simulink model "AIM_OneAgent"  (R2022b)
settings: Solver=ode4  StartTime=0.0  StopTime=inf  FixedStep=0.01  RelTol=1e-3
libraries: simulink x6, slpidlib x4, sim3dautolib x4, rllib x2, sim3dlib x1
(part 1 of 2)
settings Model: Creator=DELL G3  LastModifiedBy=DELL G3
settings DebuggingCC: IgnoredZcDiagnostic=none

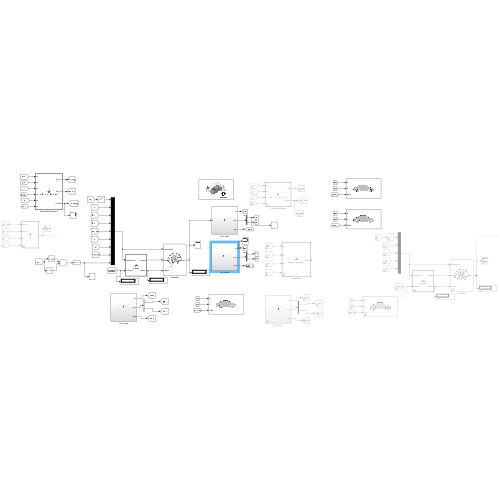
[thumbnail: Simulink's stored preview of the top-level diagram]
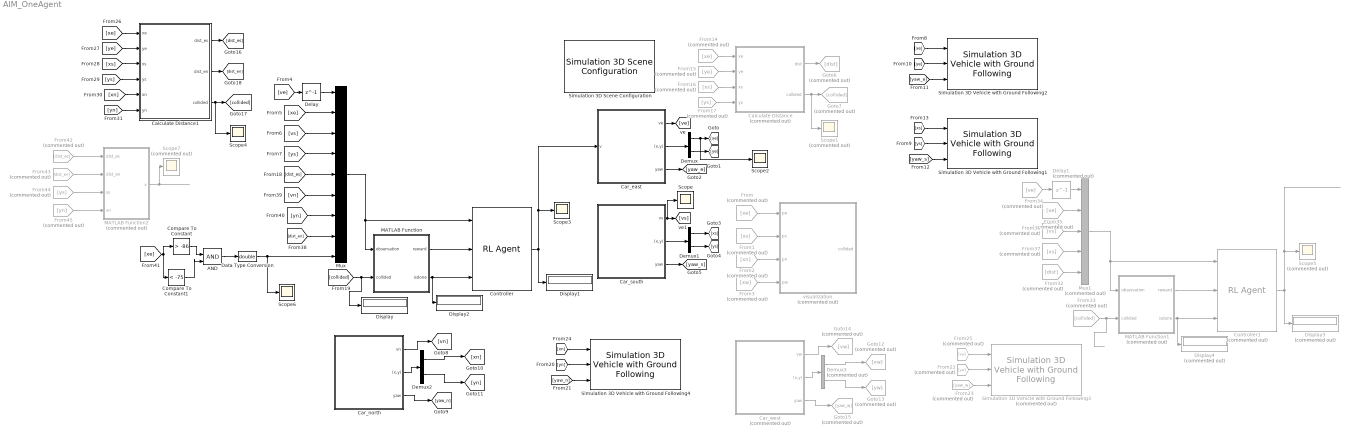
== system AIM_OneAgent ==
  AND : Logic  IconShape=distinctive  AllPortsSameDT=off  OutDataTypeStr=boolean
  Calculate Distance : MATLAB Function  Commented=on  TreatAsAtomicUnit=on
  Calculate Distance1 : MATLAB Function  TreatAsAtomicUnit=on
  Car_east : Subsystem
  Car_north : Subsystem
  Car_south : Subsystem
  Car_west : Subsystem  Commented=on
  Compare To Constant : simulink/Logic and Bit Operations/Compare To Constant  relop=>  const=-86  OutDataTypeStr=boolean
  Compare To Constant1 : simulink/Logic and Bit Operations/Compare To Constant  relop=<  const=-75  OutDataTypeStr=boolean
  Controller : rllib/RL Agent  Agent=car_agent_Trained  ExternalActionAsInput=off  ProvideLastAction=off  ProvideCumRwd=off  TreatAsDirectFeedthrough=on  UseStrictObservationDataTypes=off
  Controller1 : rllib/RL Agent  Commented=on  Agent=agent1_Trained_Trained  ExternalActionAsInput=off  ProvideLastAction=off  ProvideCumRwd=off  TreatAsDirectFeedthrough=on  UseStrictObservationDataTypes=off
  Data Type Conversion : DataTypeConversion  OutDataTypeStr=double  SaturateOnIntegerOverflow=off  RndMeth=Floor
  Delay : Delay  DelayLength=1
  Delay1 : Delay  Commented=on  DelayLength=1
  Demux : Demux  Outputs=2
  Demux1 : Demux  Outputs=2
  Demux2 : Demux  Outputs=2
  Demux3 : Demux  Commented=on  Outputs=2
  Display : Display
  Display1 : Display
  Display2 : Display
  Display3 : Display  Commented=on
  Display4 : Display  Commented=on
  From : From  Commented=on  GotoTag=xe
  From1 : From  Commented=on  GotoTag=xs
  From14 : From  Commented=on  GotoTag=xe
  From15 : From  Commented=on  GotoTag=ye
  From16 : From  Commented=on  GotoTag=xs
  From17 : From  Commented=on  GotoTag=ys
  From2 : From  Commented=on  GotoTag=xn
  From22 : From  Commented=on  GotoTag=yw
  From23 : From  Commented=on  GotoTag=yaw_w
  From25 : From  Commented=on  GotoTag=xw
  From3 : From  Commented=on  GotoTag=xw
  From32 : From  Commented=on  GotoTag=dist
  From33 : From  Commented=on  GotoTag=collided
  From34 : From  Commented=on  GotoTag=ve
  From35 : From  Commented=on  GotoTag=xe
  From36 : From  Commented=on  GotoTag=vs
  From37 : From  Commented=on  GotoTag=xs
  From42 : From  Commented=on  GotoTag=dist_es
  From43 : From  Commented=on  GotoTag=dist_en
  From44 : From  Commented=on  GotoTag=ys
  From45 : From  Commented=on  GotoTag=yn
  Goto12 : Goto  Commented=on  GotoTag=xw
  Goto13 : Goto  Commented=on  GotoTag=yw
  Goto14 : Goto  Commented=on  GotoTag=vw
  Goto15 : Goto  Commented=on  GotoTag=yaw_w
  Goto6 : Goto  Commented=on  GotoTag=dist
  Goto7 : Goto  Commented=on  GotoTag=collided
  MATLAB Function : MATLAB Function  TreatAsAtomicUnit=on
  MATLAB Function1 : MATLAB Function  Commented=on  TreatAsAtomicUnit=on
  MATLAB Function2 : MATLAB Function  Commented=on  TreatAsAtomicUnit=on
  Mux : Mux  Inputs=9
  Mux1 : Mux  Commented=on  Inputs=5
  Scope{,2..4,6} (5 alike) : Scope
  Scope1 : Scope  Commented=on
  Scope5 : Scope  Commented=on
  Scope7 : Scope  Commented=on
  Simulation 3D Scene Configuration : sim3dlib/Simulation 3D Scene Configuration  Priority=0  ProjectFormat=Default Scenes  SceneDesc=US city block  ProjectName=C:\Program Files\MATLAB\R2022b\toolbox\shared\sim3d_projects\automotive_project\UE4\WindowsNoEditor\VehicleSimulation.exe  ScenePath=/Game/Maps/HwStrght  EnableOpenDRIVE=off  vehTagList={'Scene Origin';'car_east';'car_north';'car_south';'car_west'}  vehTag=car_east  OpVisEn=off  Ts=0.01  EnableWindow=on  EnableRemoteAccess=off  EnableWeather=off  SunAltitude=40.0  SunAzimuth=90  clouds=10  wind=1  fog=0  rain=0  EnableGeospatial=off  OriginHeight=200  OriginLatitude=40.744652  OriginLongitude=-73.988864  MapStyle=Aerial  AdditionalAssetIDs=[]  UseAdvancedSunSky=off  SolarTime=11  TimeZone=-5  Day=21  Month=9  Year=2022  UseDaylightSavingTime=on  DSTStartDay=10  DSTStartMonth=3  DSTEndDay=3  DSTEndMonth=11  DSTSwitchHour=2  sensorTag=MainCamera1  sensorId=1  sensorName=MainCamera1  mountLoc=Origin  offsetFlag=off  tmountOffset=[0, 0, 0]  rmountOffset=[0, 0, 0]  HorizontalResolution=1280  VerticalResolution=720  HorizontalFOV=60  mountPoint=[0 0 0]  mountOrientation=[0 0 0]  aMode=3  ID=1  GeoTrigger=Inactive
      settings: LibrarySourceBlock=drivingsim3d/Simulation 3D Scene Configuration
  Simulation 3D Vehicle with Ground Following1 : sim3dautolib/Simulation 3D Vehicle with Ground Following  Priority=-1  PassVehMesh=Muscle car  MeshPath=/MathWorksAutomotiveContent/Vehicles/Muscle/Meshes/SK_MuscleCar.SK_MuscleCar  TrackWidth=1.9  WheelBase=3  WheelRadius=0.35  VehColor=Yellow  InitialPos=[0, 0, 0]  InitialRot=[0, 0, 0]  ActorName=car_south  SampleTime=-1  ActorType=SimulinkVehicle  ID=C  aMode=3  ActorTag=car_south  CoordinateScheme=ISO  VehLightsControl=off  HeadlightColor=[ 1, 1, 1 ]  HighBeamIntensity=100000  LowBeamIntensity=60000  HighBeamConeAngle=70  LowBeamConeAngle=70  LeftHeadlightOrientation=[ 0, 0 ]  RightHeadlightOrientation=[ 0, 0 ]  BrakelightIntensity=500  ReverselightIntensity=500  SignallightIntensity=500  SignallightPeriod=1  SignalPulseWidth=50  TransformOutportEnabled=off
      settings: LibrarySourceBlock=drivingsim3d/Simulation 3D Vehicle with Ground Following
  Simulation 3D Vehicle with Ground Following2 : sim3dautolib/Simulation 3D Vehicle with Ground Following  Priority=-1  PassVehMesh=Muscle car  MeshPath=/MathWorksAutomotiveContent/Vehicles/Muscle/Meshes/SK_MuscleCar.SK_MuscleCar  TrackWidth=1.9  WheelBase=3  WheelRadius=0.35  VehColor=Red  InitialPos=[0, 0, 0]  InitialRot=[0, 0, 0]  ActorName=car_east  SampleTime=-1  ActorType=SimulinkVehicle  ID=C  aMode=3  ActorTag=car_east  CoordinateScheme=ISO  VehLightsControl=off  HeadlightColor=[ 1, 1, 1 ]  HighBeamIntensity=100000  LowBeamIntensity=60000  HighBeamConeAngle=70  LowBeamConeAngle=70  LeftHeadlightOrientation=[ 0, 0 ]  RightHeadlightOrientation=[ 0, 0 ]  BrakelightIntensity=500  ReverselightIntensity=500  SignallightIntensity=500  SignallightPeriod=1  SignalPulseWidth=50  TransformOutportEnabled=off
      settings: LibrarySourceBlock=drivingsim3d/Simulation 3D Vehicle with Ground Following
  Simulation 3D Vehicle with Ground Following3 : sim3dautolib/Simulation 3D Vehicle with Ground Following  Priority=-1  Commented=on  PassVehMesh=Muscle car  MeshPath=/MathWorksAutomotiveContent/Vehicles/Muscle/Meshes/SK_MuscleCar.SK_MuscleCar  TrackWidth=1.9  WheelBase=3  WheelRadius=0.35  VehColor=Green  InitialPos=[0, 0, 0]  InitialRot=[0, 0, 0]  ActorName=car_west  SampleTime=-1  ActorType=SimulinkVehicle  ID=C  aMode=3  ActorTag=car_west  CoordinateScheme=ISO  VehLightsControl=off  HeadlightColor=[ 1, 1, 1 ]  HighBeamIntensity=100000  LowBeamIntensity=60000  HighBeamConeAngle=70  LowBeamConeAngle=70  LeftHeadlightOrientation=[ 0, 0 ]  RightHeadlightOrientation=[ 0, 0 ]  BrakelightIntensity=500  ReverselightIntensity=500  SignallightIntensity=500  SignallightPeriod=1  SignalPulseWidth=50  TransformOutportEnabled=off
      settings: LibrarySourceBlock=drivingsim3d/Simulation 3D Vehicle with Ground Following
  Simulation 3D Vehicle with Ground Following4 : sim3dautolib/Simulation 3D Vehicle with Ground Following  Priority=-1  PassVehMesh=Muscle car  MeshPath=/MathWorksAutomotiveContent/Vehicles/Muscle/Meshes/SK_MuscleCar.SK_MuscleCar  TrackWidth=1.9  WheelBase=3  WheelRadius=0.35  VehColor=Blue  InitialPos=[0, 0, 0]  InitialRot=[0, 0, 0]  ActorName=car_north  SampleTime=-1  ActorType=SimulinkVehicle  ID=C  aMode=3  ActorTag=car_north  CoordinateScheme=ISO  VehLightsControl=off  HeadlightColor=[ 1, 1, 1 ]  HighBeamIntensity=100000  LowBeamIntensity=60000  HighBeamConeAngle=70  LowBeamConeAngle=70  LeftHeadlightOrientation=[ 0, 0 ]  RightHeadlightOrientation=[ 0, 0 ]  BrakelightIntensity=500  ReverselightIntensity=500  SignallightIntensity=500  SignallightPeriod=1  SignalPulseWidth=50  TransformOutportEnabled=off
      settings: LibrarySourceBlock=drivingsim3d/Simulation 3D Vehicle with Ground Following
  visualization : MATLAB Function  Commented=on  TreatAsAtomicUnit=on
  wires:
  MATLAB Function/1(reward) -> Controller/2
  MATLAB Function/2(isdone) -> Controller/3, Display2/1
  Car_east/1(ve) -> [ve]
  From/1 -> visualization/1(pe)
  From1/1 -> visualization/2(ps)
  From2/1 -> visualization/3(pn)
  From3/1 -> visualization/4(pw)
  [ve] -> Delay/1
  [xe] -> Mux/2
  [vs] -> Mux/3
  [ys] -> Mux/4
  Mux/1 -> Controller/1, MATLAB Function/1(observation)
  Car_east/2((x,y)) -> Demux/1
  Demux/1 -> Scope2/1, [xe]
  Demux/2 -> [ye]
  Car_east/3(yaw) -> [yaw_e]
  [ye] -> Simulation 3D Vehicle with Ground Following2/2
  [yaw_e] -> Simulation 3D Vehicle with Ground Following2/3
  Demux1/1 -> [xs]
  Demux1/2 -> [ys]
  Car_south/3(yaw) -> [yaw_s]
  Car_south/2((x,y)) -> Demux1/1
  Car_south/1(vs) -> Scope/1, [vs]
  [yaw_s] -> Simulation 3D Vehicle with Ground Following1/3
  [xs] -> Simulation 3D Vehicle with Ground Following1/1
  From14/1 -> Calculate Distance/1(xe)
  From15/1 -> Calculate Distance/2(ye)
  From16/1 -> Calculate Distance/3(xs)
  From17/1 -> Calculate Distance/4(ys)
  Calculate Distance/1(dist) -> Goto6/1
  [xe] -> Simulation 3D Vehicle with Ground Following2/1
  [ys] -> Simulation 3D Vehicle with Ground Following1/2
  [dist_es] -> Mux/5
  Calculate Distance/2(collided) -> Scope1/1, Goto7/1
  [collided] -> Display/1, MATLAB Function/2(collided)
  [yn] -> Simulation 3D Vehicle with Ground Following4/2
  [yaw_n] -> Simulation 3D Vehicle with Ground Following4/3
  [xn] -> Simulation 3D Vehicle with Ground Following4/1
  Demux2/1 -> [xn]
  Car_north/1(vn) -> [vn]
  Car_north/3(yaw) -> [yaw_n]
  Demux2/2 -> [yn]
  Car_north/2((x,y)) -> Demux2/1
  Car_west/2((x,y)) -> Demux3/1
  From25/1 -> Simulation 3D Vehicle with Ground Following3/1
  Car_west/3(yaw) -> Goto15/1
  Demux3/1 -> Goto12/1
  Demux3/2 -> Goto13/1
  Car_west/1(vw) -> Goto14/1
  From23/1 -> Simulation 3D Vehicle with Ground Following3/3
  From22/1 -> Simulation 3D Vehicle with Ground Following3/2
  Delay/1 -> Mux/1
  [xs] -> Calculate Distance1/3(xs)
  Calculate Distance1/3(collided) -> [collided], Scope4/1
  Calculate Distance1/1(dist_es) -> [dist_es]
  [xe] -> Calculate Distance1/1(xe)
  [ys] -> Calculate Distance1/4(ys)
  [ye] -> Calculate Distance1/2(ye)
  [xn] -> Calculate Distance1/5(xn)
  [yn] -> Calculate Distance1/6(yn)
  Calculate Distance1/2(dist_en) -> [dist_en]
  Delay1/1 -> Mux1/1
  From35/1 -> Mux1/2
  Controller1/1 -> Display3/1, Scope5/1
  MATLAB Function1/2(isdone) -> Controller1/3, Display4/1
  Mux1/1 -> Controller1/1, MATLAB Function1/1(observation)
  From37/1 -> Mux1/4
  From33/1 -> MATLAB Function1/2(collided)
  From34/1 -> Delay1/1
  From36/1 -> Mux1/3
  MATLAB Function1/1(reward) -> Controller1/2
  From32/1 -> Mux1/5
  [yn] -> Mux/7
  [vn] -> Mux/6
  [dist_en] -> Mux/8
  [xe] -> Compare To Constant1/1, Compare To Constant/1
  Compare To Constant1/1 -> AND/2
  AND/1 -> Data Type Conversion/1
  Compare To Constant/1 -> AND/1
  Data Type Conversion/1 -> Mux/9, Scope6/1
  Controller/1 -> Car_east/1(v), Scope3/1, Display1/1
  From42/1 -> MATLAB Function2/1(dist_es)
  From43/1 -> MATLAB Function2/2(dist_en)
  MATLAB Function2/1(v) -> Scope7/1
  From44/1 -> MATLAB Function2/3(xs)
  From45/1 -> MATLAB Function2/4(xn)

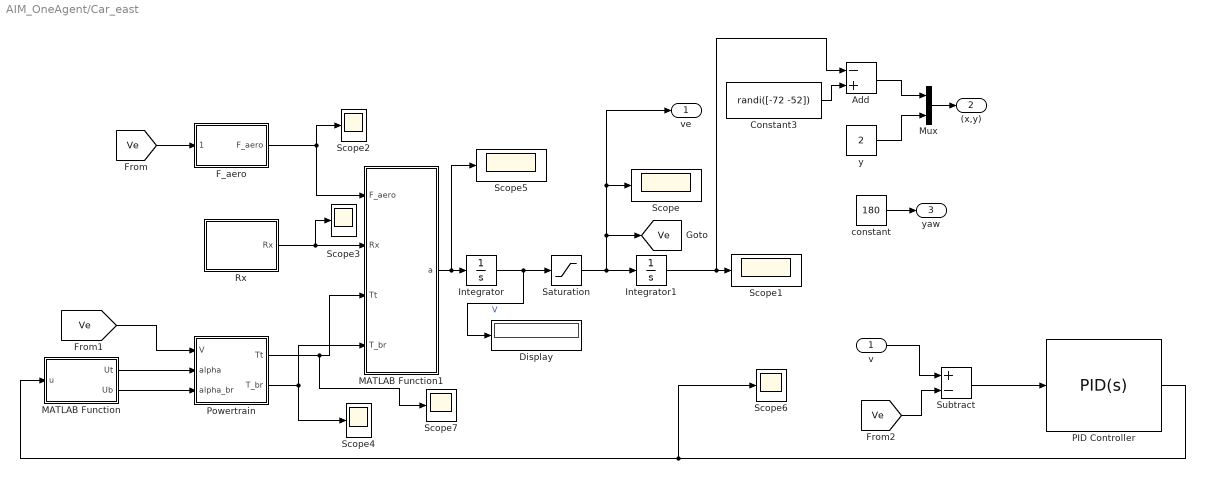
== system AIM_OneAgent/Car_east ==
  v : Inport
  Add : Sum  Inputs=-+
  Constant3 : Constant  Value=randi([-72 -52])
  Display : Display
  F_aero : Subsystem
  Integrator : Integrator
  Integrator1 : Integrator
  MATLAB Function : MATLAB Function  TreatAsAtomicUnit=on
  MATLAB Function1 : MATLAB Function  TreatAsAtomicUnit=on
  Mux : Mux  Inputs=2
  PID Controller : slpidlib/PID Controller  Controller=PID  Form=Parallel  TimeDomain=Continuous-time  UseExternalTs=off  SampleTime=-1  IntegratorMethod=Forward Euler  FilterMethod=Forward Euler  ControllerParametersSource=internal  P=1000  I=5  UseKiTs=off  D=0  N=100  UseFilter=on  TunerSelectOption=Transfer Function Based (PID Tuner App)  InitialConditionSource=internal  InitialConditionForIntegrator=0  InitialConditionForFilter=0  DifferentiatorICPrevScaledInput=0  ExternalReset=none  TrackingMode=off  Kt=1  LimitOutput=on  SatLimitsSource=internal  UpperSaturationLimit=1  LowerSaturationLimit=-1  LinearizeAsGain=on  AntiWindupMode=none  Kb=1  LimitIntegrator=off  UpperIntegratorSaturationLimit=inf  LowerIntegratorSaturationLimit=-inf  POutMin=[]  POutMax=[]  IOutMin=[]  IOutMax=[]  DOutMin=[]  DOutMax=[]  NOutMin=[]  NOutMax=[]  SumOutMin=[]  SumOutMax=[]  SaturationOutMin=[]  SaturationOutMax=[]  PParamMin=[]  PParamMax=[]  IParamMin=[]  IParamMax=[]  DParamMin=[]  DParamMax=[]  NParamMin=[]  NParamMax=[]  KbParamMin=[]  KbParamMax=[]  KtParamMin=[]  KtParamMax=[]  KbOutMin=[]  KbOutMax=[]  KtOutMin=[]  KtOutMax=[]  IntegratorOutMin=[]  IntegratorOutMax=[]  FilterOutMin=[]  FilterOutMax=[]  SumI1OutMin=[]  SumI1OutMax=[]  SumI2OutMin=[]  SumI2OutMax=[]  SumI3OutMin=[]  SumI3OutMax=[]  SumI4OutMin=[]  SumI4OutMax=[]  SumDOutMin=[]  SumDOutMax=[]  DifferentiatorOutMin=[]  DifferentiatorOutMax=[]  FilterDiffOutCoefMin=[]  FilterDiffOutCoefMax=[]  ReciprocalOutMin=[]  ReciprocalOutMax=[]  SumDenOutMin=[]  SumDenOutMax=[]  SumNumOutMin=[]  SumNumOutMax=[]  DivideOutMin=[]  DivideOutMax=[]  UdiffTsProdOutMin=[]  UdiffTsProdOutMax=[]  NTsProdOutMin=[]  NTsProdOutMax=[]  UintegralTsProdOutMin=[]  UintegralTsProdOutMax=[]  UngainTsProdOutMin=[]  UngainTsProdOutMax=[]  ClampingZeroOutDataTypeStr=Inherit: Inherit via back propagation  ClampingZeroOutMin=[]  ClampingZeroOutMax=[]  FilterDenConstantOutDataTypeStr=Inherit: Inherit via back propagation  FilterDenConstantOutMin=[]  FilterDenConstantOutMax=[]  PCopyOutDataTypeStr=Inherit: Inherit via back propagation  PCopyOutMin=[]  PCopyOutMax=[]  NCopyOutDataTypeStr=Inherit: Inherit via back propagation  NCopyOutMin=[]  NCopyOutMax=[]  IntegratorContinuousStateAttributes=''  IntegratorStateMustResolveToSignalObject=off  IntegratorRTWStateStorageClass=Auto  FilterContinuousStateAttributes=''  FilterStateMustResolveToSignalObject=off  FilterRTWStateStorageClass=Auto  ParallelPVariant=InternalParameters  IdealPVariant=Disabled  IVariant=InternalParameters  DVariant=InternalParameters  IntegratorVariant=Continuous  SatVariant=Enabled  AWVariant=Passthrough  PCopyVariant=Disabled  TRVariant=Disabled  FdbkBlocksVariant=Forward  IdealPFdbkVariant=Disabled  SatFdbkVariant=Disabled  DerivativeFilterVariant=ContFilter  NVariant=InternalParameters  NCopyVariant=Disabled  FilterICVariant=InternalICsFilter  IntegratorICVariant=InternalICs  ExternalResetVariant=Disabled  TRSumVariant=Passthrough  SumFdbkVariant=Disabled  SumVariant=Sum_PID  TsampFilterVariant=InternalTs  TsampNgainVariant=Passthrough  TsampIntegralVariant=Passthrough  ExternalSaturationOutDataTypeStr=Inherit: Same as second input
  Powertrain : Subsystem
  Rx : Subsystem
  Saturation : Saturate  UpperLimit=25  LowerLimit=0
  Scope{,1..7} (8 alike) : Scope
  Subtract : Sum  Inputs=+-
  constant : Constant  Value=180
  y : Constant  Value=2
  ve : Outport
  (x,y) : Outport  Port=2
  yaw : Outport  Port=3
  tag scope: Ve=global
  wires:
  Rx/1(Rx) -> Scope3/1, MATLAB Function1/2(Rx)
  F_aero/1(F_aero) -> MATLAB Function1/1(F_aero), Scope2/1
  [Ve] -> F_aero/1(velocity)
  PID Controller/1 -> Scope6/1, MATLAB Function/1(u)
  Saturation/1 -> ve/1, Scope/1, [Ve], Integrator1/1
  Powertrain/1(Tt) -> Scope7/1, MATLAB Function1/3(Tt)
  Integrator/1 -> Saturation/1, Display/1  "V"
  MATLAB Function1/1(a) -> Scope5/1, Integrator/1
  [Ve] -> Subtract/2
  [Ve] -> Powertrain/1(V)
  Powertrain/2(T_br) -> Scope4/1, MATLAB Function1/4(T_br)
  Subtract/1 -> PID Controller/1
  v/1 -> Subtract/1
  MATLAB Function/1(Ut) -> Powertrain/2(alpha)
  MATLAB Function/2(Ub) -> Powertrain/3(alpha_br)
  y/1 -> Mux/2
  Mux/1 -> (x,y)/1
  constant/1 -> yaw/1
  Integrator1/1 -> Add/1, Scope1/1
  Constant3/1 -> Add/2
  Add/1 -> Mux/1

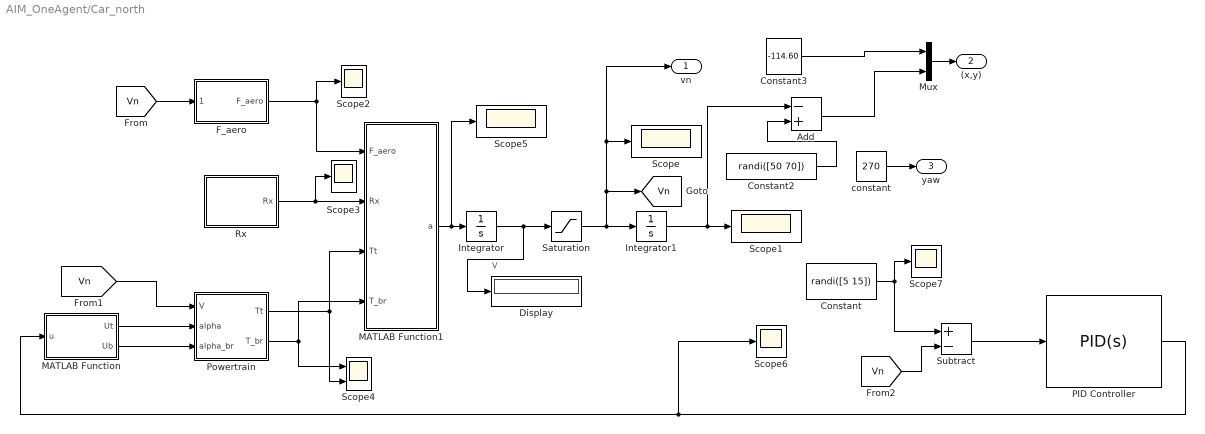
== system AIM_OneAgent/Car_north ==
  Add : Sum  Inputs=-+
  Constant : Constant  Value=randi([5 15])
  Constant2 : Constant  Value=randi([50 70])
  Constant3 : Constant  Value=-114.60
  Display : Display
  F_aero : Subsystem
  Integrator : Integrator
  Integrator1 : Integrator
  MATLAB Function : MATLAB Function  TreatAsAtomicUnit=on
  MATLAB Function1 : MATLAB Function  TreatAsAtomicUnit=on
  Mux : Mux  Inputs=2
  PID Controller : slpidlib/PID Controller  Controller=PID  Form=Parallel  TimeDomain=Continuous-time  UseExternalTs=off  SampleTime=-1  IntegratorMethod=Forward Euler  FilterMethod=Forward Euler  ControllerParametersSource=internal  P=1000  I=5  UseKiTs=off  D=0  N=100  UseFilter=on  TunerSelectOption=Transfer Function Based (PID Tuner App)  InitialConditionSource=internal  InitialConditionForIntegrator=0  InitialConditionForFilter=0  DifferentiatorICPrevScaledInput=0  ExternalReset=none  TrackingMode=off  Kt=1  LimitOutput=on  SatLimitsSource=internal  UpperSaturationLimit=1  LowerSaturationLimit=-1  LinearizeAsGain=on  AntiWindupMode=none  Kb=1  LimitIntegrator=off  UpperIntegratorSaturationLimit=inf  LowerIntegratorSaturationLimit=-inf  POutMin=[]  POutMax=[]  IOutMin=[]  IOutMax=[]  DOutMin=[]  DOutMax=[]  NOutMin=[]  NOutMax=[]  SumOutMin=[]  SumOutMax=[]  SaturationOutMin=[]  SaturationOutMax=[]  PParamMin=[]  PParamMax=[]  IParamMin=[]  IParamMax=[]  DParamMin=[]  DParamMax=[]  NParamMin=[]  NParamMax=[]  KbParamMin=[]  KbParamMax=[]  KtParamMin=[]  KtParamMax=[]  KbOutMin=[]  KbOutMax=[]  KtOutMin=[]  KtOutMax=[]  IntegratorOutMin=[]  IntegratorOutMax=[]  FilterOutMin=[]  FilterOutMax=[]  SumI1OutMin=[]  SumI1OutMax=[]  SumI2OutMin=[]  SumI2OutMax=[]  SumI3OutMin=[]  SumI3OutMax=[]  SumI4OutMin=[]  SumI4OutMax=[]  SumDOutMin=[]  SumDOutMax=[]  DifferentiatorOutMin=[]  DifferentiatorOutMax=[]  FilterDiffOutCoefMin=[]  FilterDiffOutCoefMax=[]  ReciprocalOutMin=[]  ReciprocalOutMax=[]  SumDenOutMin=[]  SumDenOutMax=[]  SumNumOutMin=[]  SumNumOutMax=[]  DivideOutMin=[]  DivideOutMax=[]  UdiffTsProdOutMin=[]  UdiffTsProdOutMax=[]  NTsProdOutMin=[]  NTsProdOutMax=[]  UintegralTsProdOutMin=[]  UintegralTsProdOutMax=[]  UngainTsProdOutMin=[]  UngainTsProdOutMax=[]  ClampingZeroOutDataTypeStr=Inherit: Inherit via back propagation  ClampingZeroOutMin=[]  ClampingZeroOutMax=[]  FilterDenConstantOutDataTypeStr=Inherit: Inherit via back propagation  FilterDenConstantOutMin=[]  FilterDenConstantOutMax=[]  PCopyOutDataTypeStr=Inherit: Inherit via back propagation  PCopyOutMin=[]  PCopyOutMax=[]  NCopyOutDataTypeStr=Inherit: Inherit via back propagation  NCopyOutMin=[]  NCopyOutMax=[]  IntegratorContinuousStateAttributes=''  IntegratorStateMustResolveToSignalObject=off  IntegratorRTWStateStorageClass=Auto  FilterContinuousStateAttributes=''  FilterStateMustResolveToSignalObject=off  FilterRTWStateStorageClass=Auto  ParallelPVariant=InternalParameters  IdealPVariant=Disabled  IVariant=InternalParameters  DVariant=InternalParameters  IntegratorVariant=Continuous  SatVariant=Enabled  AWVariant=Passthrough  PCopyVariant=Disabled  TRVariant=Disabled  FdbkBlocksVariant=Forward  IdealPFdbkVariant=Disabled  SatFdbkVariant=Disabled  DerivativeFilterVariant=ContFilter  NVariant=InternalParameters  NCopyVariant=Disabled  FilterICVariant=InternalICsFilter  IntegratorICVariant=InternalICs  ExternalResetVariant=Disabled  TRSumVariant=Passthrough  SumFdbkVariant=Disabled  SumVariant=Sum_PID  TsampFilterVariant=InternalTs  TsampNgainVariant=Passthrough  TsampIntegralVariant=Passthrough  ExternalSaturationOutDataTypeStr=Inherit: Same as second input
  Powertrain : Subsystem
  Rx : Subsystem
  Saturation : Saturate  UpperLimit=25  LowerLimit=0
  Scope{,1..3,5..7} (7 alike) : Scope
  Scope4 : Scope  NumInputPorts=2
  Subtract : Sum  Inputs=+-
  constant : Constant  Value=270
  vn : Outport
  (x,y) : Outport  Port=2
  yaw : Outport  Port=3
  tag scope: Vn=global
  wires:
  Rx/1(Rx) -> Scope3/1, MATLAB Function1/2(Rx)
  F_aero/1(F_aero) -> MATLAB Function1/1(F_aero), Scope2/1
  [Vn] -> F_aero/1(velocity)
  PID Controller/1 -> Scope6/1, MATLAB Function/1(u)
  Saturation/1 -> vn/1, Scope/1, [Vn], Integrator1/1
  Powertrain/1(Tt) -> Scope4/2, MATLAB Function1/3(Tt)
  Integrator/1 -> Saturation/1, Display/1  "V"
  MATLAB Function1/1(a) -> Scope5/1, Integrator/1
  [Vn] -> Subtract/2
  [Vn] -> Powertrain/1(V)
  Powertrain/2(T_br) -> Scope4/1, MATLAB Function1/4(T_br)
  Subtract/1 -> PID Controller/1
  MATLAB Function/1(Ut) -> Powertrain/2(alpha)
  MATLAB Function/2(Ub) -> Powertrain/3(alpha_br)
  Mux/1 -> (x,y)/1
  constant/1 -> yaw/1
  Integrator1/1 -> Add/1, Scope1/1
  Constant3/1 -> Mux/1
  Add/1 -> Mux/2
  Constant2/1 -> Add/2
  Constant/1 -> Subtract/1, Scope7/1

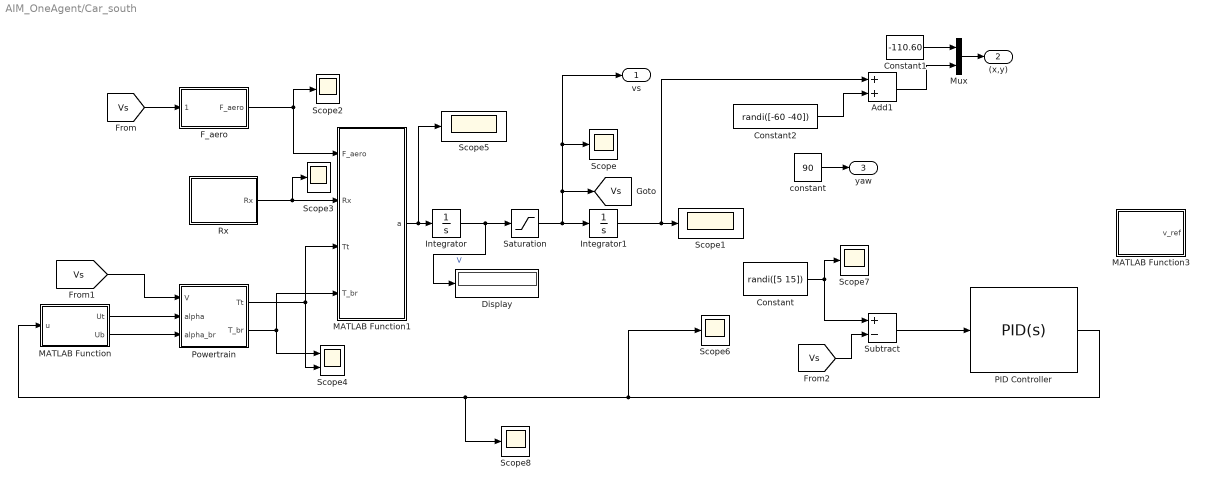
== system AIM_OneAgent/Car_south ==
  Add1 : Sum
  Constant : Constant  Value=randi([5 15])
  Constant1 : Constant  Value=-110.60
  Constant2 : Constant  Value=randi([-60 -40])
  Display : Display
  F_aero : Subsystem
  Integrator : Integrator
  Integrator1 : Integrator
  MATLAB Function : MATLAB Function  TreatAsAtomicUnit=on
  MATLAB Function1 : MATLAB Function  TreatAsAtomicUnit=on
  MATLAB Function3 : MATLAB Function  TreatAsAtomicUnit=on
  Mux : Mux  Inputs=2
  PID Controller : slpidlib/PID Controller  Controller=PID  Form=Parallel  TimeDomain=Continuous-time  UseExternalTs=off  SampleTime=-1  IntegratorMethod=Forward Euler  FilterMethod=Forward Euler  ControllerParametersSource=internal  P=1000  I=5  UseKiTs=off  D=0  N=100  UseFilter=on  TunerSelectOption=Transfer Function Based (PID Tuner App)  InitialConditionSource=internal  InitialConditionForIntegrator=0  InitialConditionForFilter=0  DifferentiatorICPrevScaledInput=0  ExternalReset=none  TrackingMode=off  Kt=1  LimitOutput=on  SatLimitsSource=internal  UpperSaturationLimit=1  LowerSaturationLimit=-1  LinearizeAsGain=on  AntiWindupMode=none  Kb=1  LimitIntegrator=off  UpperIntegratorSaturationLimit=inf  LowerIntegratorSaturationLimit=-inf  POutMin=[]  POutMax=[]  IOutMin=[]  IOutMax=[]  DOutMin=[]  DOutMax=[]  NOutMin=[]  NOutMax=[]  SumOutMin=[]  SumOutMax=[]  SaturationOutMin=[]  SaturationOutMax=[]  PParamMin=[]  PParamMax=[]  IParamMin=[]  IParamMax=[]  DParamMin=[]  DParamMax=[]  NParamMin=[]  NParamMax=[]  KbParamMin=[]  KbParamMax=[]  KtParamMin=[]  KtParamMax=[]  KbOutMin=[]  KbOutMax=[]  KtOutMin=[]  KtOutMax=[]  IntegratorOutMin=[]  IntegratorOutMax=[]  FilterOutMin=[]  FilterOutMax=[]  SumI1OutMin=[]  SumI1OutMax=[]  SumI2OutMin=[]  SumI2OutMax=[]  SumI3OutMin=[]  SumI3OutMax=[]  SumI4OutMin=[]  SumI4OutMax=[]  SumDOutMin=[]  SumDOutMax=[]  DifferentiatorOutMin=[]  DifferentiatorOutMax=[]  FilterDiffOutCoefMin=[]  FilterDiffOutCoefMax=[]  ReciprocalOutMin=[]  ReciprocalOutMax=[]  SumDenOutMin=[]  SumDenOutMax=[]  SumNumOutMin=[]  SumNumOutMax=[]  DivideOutMin=[]  DivideOutMax=[]  UdiffTsProdOutMin=[]  UdiffTsProdOutMax=[]  NTsProdOutMin=[]  NTsProdOutMax=[]  UintegralTsProdOutMin=[]  UintegralTsProdOutMax=[]  UngainTsProdOutMin=[]  UngainTsProdOutMax=[]  ClampingZeroOutDataTypeStr=Inherit: Inherit via back propagation  ClampingZeroOutMin=[]  ClampingZeroOutMax=[]  FilterDenConstantOutDataTypeStr=Inherit: Inherit via back propagation  FilterDenConstantOutMin=[]  FilterDenConstantOutMax=[]  PCopyOutDataTypeStr=Inherit: Inherit via back propagation  PCopyOutMin=[]  PCopyOutMax=[]  NCopyOutDataTypeStr=Inherit: Inherit via back propagation  NCopyOutMin=[]  NCopyOutMax=[]  IntegratorContinuousStateAttributes=''  IntegratorStateMustResolveToSignalObject=off  IntegratorRTWStateStorageClass=Auto  FilterContinuousStateAttributes=''  FilterStateMustResolveToSignalObject=off  FilterRTWStateStorageClass=Auto  ParallelPVariant=InternalParameters  IdealPVariant=Disabled  IVariant=InternalParameters  DVariant=InternalParameters  IntegratorVariant=Continuous  SatVariant=Enabled  AWVariant=Passthrough  PCopyVariant=Disabled  TRVariant=Disabled  FdbkBlocksVariant=Forward  IdealPFdbkVariant=Disabled  SatFdbkVariant=Disabled  DerivativeFilterVariant=ContFilter  NVariant=InternalParameters  NCopyVariant=Disabled  FilterICVariant=InternalICsFilter  IntegratorICVariant=InternalICs  ExternalResetVariant=Disabled  TRSumVariant=Passthrough  SumFdbkVariant=Disabled  SumVariant=Sum_PID  TsampFilterVariant=InternalTs  TsampNgainVariant=Passthrough  TsampIntegralVariant=Passthrough  ExternalSaturationOutDataTypeStr=Inherit: Same as second input
  Powertrain : Subsystem
  Rx : Subsystem
  Saturation : Saturate  UpperLimit=25  LowerLimit=0
  Scope{,1..3,5..8} (8 alike) : Scope
  Scope4 : Scope  NumInputPorts=2
  Subtract : Sum  Inputs=+-
  constant : Constant  Value=90
  vs : Outport
  (x,y) : Outport  Port=2
  yaw : Outport  Port=3
  tag scope: Vs=global
  wires:
  Rx/1(Rx) -> Scope3/1, MATLAB Function1/2(Rx)
  F_aero/1(F_aero) -> MATLAB Function1/1(F_aero), Scope2/1
  [Vs] -> F_aero/1(velocity)
  PID Controller/1 -> Scope6/1, Scope8/1, MATLAB Function/1(u)
  Saturation/1 -> Scope/1, vs/1, [Vs], Integrator1/1
  Powertrain/1(Tt) -> Scope4/2, MATLAB Function1/3(Tt)
  Integrator/1 -> Saturation/1, Display/1  "V"
  Integrator1/1 -> Add1/1, Scope1/1
  MATLAB Function1/1(a) -> Scope5/1, Integrator/1
  [Vs] -> Subtract/2
  [Vs] -> Powertrain/1(V)
  Powertrain/2(T_br) -> Scope4/1, MATLAB Function1/4(T_br)
  MATLAB Function/1(Ut) -> Powertrain/2(alpha)
  MATLAB Function/2(Ub) -> Powertrain/3(alpha_br)
  Mux/1 -> (x,y)/1
  constant/1 -> yaw/1
  Constant1/1 -> Mux/1
  Constant2/1 -> Add1/2
  Add1/1 -> Mux/2
  Subtract/1 -> PID Controller/1
  Constant/1 -> Scope7/1, Subtract/1

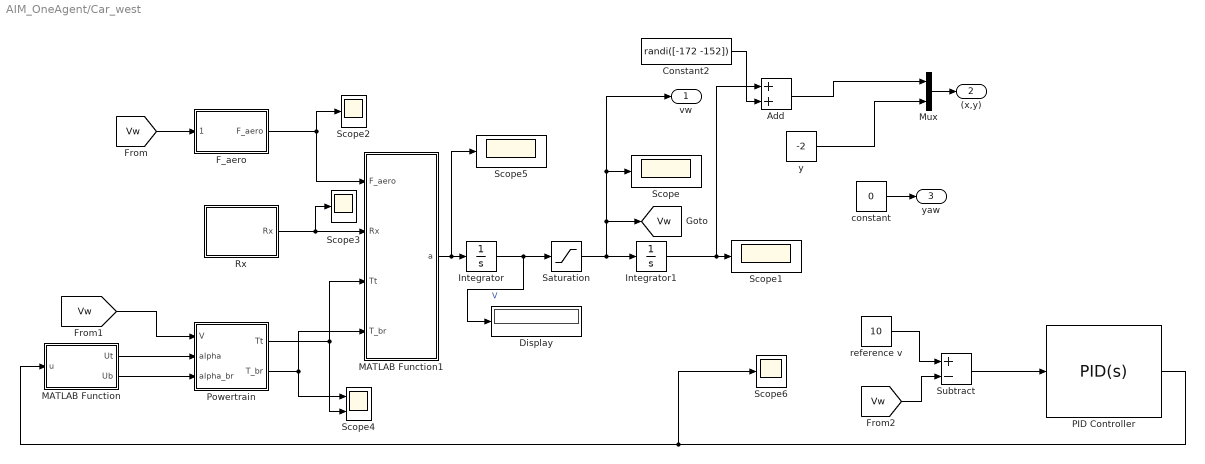
== system AIM_OneAgent/Car_west ==
  Add : Sum
  Constant2 : Constant  Value=randi([-172 -152])
  Display : Display
  F_aero : Subsystem
  Integrator : Integrator
  Integrator1 : Integrator
  MATLAB Function : MATLAB Function  TreatAsAtomicUnit=on
  MATLAB Function1 : MATLAB Function  TreatAsAtomicUnit=on
  Mux : Mux  Inputs=2
  PID Controller : slpidlib/PID Controller  Controller=PID  Form=Parallel  TimeDomain=Continuous-time  UseExternalTs=off  SampleTime=-1  IntegratorMethod=Forward Euler  FilterMethod=Forward Euler  ControllerParametersSource=internal  P=1000  I=5  UseKiTs=off  D=0  N=100  UseFilter=on  TunerSelectOption=Transfer Function Based (PID Tuner App)  InitialConditionSource=internal  InitialConditionForIntegrator=0  InitialConditionForFilter=0  DifferentiatorICPrevScaledInput=0  ExternalReset=none  TrackingMode=off  Kt=1  LimitOutput=on  SatLimitsSource=internal  UpperSaturationLimit=1  LowerSaturationLimit=-1  LinearizeAsGain=on  AntiWindupMode=none  Kb=1  LimitIntegrator=off  UpperIntegratorSaturationLimit=inf  LowerIntegratorSaturationLimit=-inf  POutMin=[]  POutMax=[]  IOutMin=[]  IOutMax=[]  DOutMin=[]  DOutMax=[]  NOutMin=[]  NOutMax=[]  SumOutMin=[]  SumOutMax=[]  SaturationOutMin=[]  SaturationOutMax=[]  PParamMin=[]  PParamMax=[]  IParamMin=[]  IParamMax=[]  DParamMin=[]  DParamMax=[]  NParamMin=[]  NParamMax=[]  KbParamMin=[]  KbParamMax=[]  KtParamMin=[]  KtParamMax=[]  KbOutMin=[]  KbOutMax=[]  KtOutMin=[]  KtOutMax=[]  IntegratorOutMin=[]  IntegratorOutMax=[]  FilterOutMin=[]  FilterOutMax=[]  SumI1OutMin=[]  SumI1OutMax=[]  SumI2OutMin=[]  SumI2OutMax=[]  SumI3OutMin=[]  SumI3OutMax=[]  SumI4OutMin=[]  SumI4OutMax=[]  SumDOutMin=[]  SumDOutMax=[]  DifferentiatorOutMin=[]  DifferentiatorOutMax=[]  FilterDiffOutCoefMin=[]  FilterDiffOutCoefMax=[]  ReciprocalOutMin=[]  ReciprocalOutMax=[]  SumDenOutMin=[]  SumDenOutMax=[]  SumNumOutMin=[]  SumNumOutMax=[]  DivideOutMin=[]  DivideOutMax=[]  UdiffTsProdOutMin=[]  UdiffTsProdOutMax=[]  NTsProdOutMin=[]  NTsProdOutMax=[]  UintegralTsProdOutMin=[]  UintegralTsProdOutMax=[]  UngainTsProdOutMin=[]  UngainTsProdOutMax=[]  ClampingZeroOutDataTypeStr=Inherit: Inherit via back propagation  ClampingZeroOutMin=[]  ClampingZeroOutMax=[]  FilterDenConstantOutDataTypeStr=Inherit: Inherit via back propagation  FilterDenConstantOutMin=[]  FilterDenConstantOutMax=[]  PCopyOutDataTypeStr=Inherit: Inherit via back propagation  PCopyOutMin=[]  PCopyOutMax=[]  NCopyOutDataTypeStr=Inherit: Inherit via back propagation  NCopyOutMin=[]  NCopyOutMax=[]  IntegratorContinuousStateAttributes=''  IntegratorStateMustResolveToSignalObject=off  IntegratorRTWStateStorageClass=Auto  FilterContinuousStateAttributes=''  FilterStateMustResolveToSignalObject=off  FilterRTWStateStorageClass=Auto  ParallelPVariant=InternalParameters  IdealPVariant=Disabled  IVariant=InternalParameters  DVariant=InternalParameters  IntegratorVariant=Continuous  SatVariant=Enabled  AWVariant=Passthrough  PCopyVariant=Disabled  TRVariant=Disabled  FdbkBlocksVariant=Forward  IdealPFdbkVariant=Disabled  SatFdbkVariant=Disabled  DerivativeFilterVariant=ContFilter  NVariant=InternalParameters  NCopyVariant=Disabled  FilterICVariant=InternalICsFilter  IntegratorICVariant=InternalICs  ExternalResetVariant=Disabled  TRSumVariant=Passthrough  SumFdbkVariant=Disabled  SumVariant=Sum_PID  TsampFilterVariant=InternalTs  TsampNgainVariant=Passthrough  TsampIntegralVariant=Passthrough  ExternalSaturationOutDataTypeStr=Inherit: Same as second input
  Powertrain : Subsystem
  Rx : Subsystem
  Saturation : Saturate  UpperLimit=25  LowerLimit=0
  Scope{,1..3,5..6} (6 alike) : Scope
  Scope4 : Scope  NumInputPorts=2
  Subtract : Sum  Inputs=+-
  constant : Constant  Value=0
  reference v : Constant  Value=10
  y : Constant  Value=-2
  vw : Outport
  (x,y) : Outport  Port=2
  yaw : Outport  Port=3
  tag scope: Vw=global
  wires:
  Rx/1(Rx) -> Scope3/1, MATLAB Function1/2(Rx)
  F_aero/1(F_aero) -> MATLAB Function1/1(F_aero), Scope2/1
  [Vw] -> F_aero/1(velocity)
  PID Controller/1 -> Scope6/1, MATLAB Function/1(u)
  Saturation/1 -> vw/1, Scope/1, [Vw], Integrator1/1
  Powertrain/1(Tt) -> Scope4/2, MATLAB Function1/3(Tt)
  Integrator/1 -> Saturation/1, Display/1  "V"
  MATLAB Function1/1(a) -> Scope5/1, Integrator/1
  [Vw] -> Subtract/2
  [Vw] -> Powertrain/1(V)
  Powertrain/2(T_br) -> Scope4/1, MATLAB Function1/4(T_br)
  Subtract/1 -> PID Controller/1
  reference v/1 -> Subtract/1
  MATLAB Function/1(Ut) -> Powertrain/2(alpha)
  MATLAB Function/2(Ub) -> Powertrain/3(alpha_br)
  Mux/1 -> (x,y)/1
  constant/1 -> yaw/1
  Integrator1/1 -> Add/1, Scope1/1
  y/1 -> Mux/2
  Add/1 -> Mux/1
  Constant2/1 -> Add/2

== system AIM_OneAgent/Car_east/F_aero ==
  velocity : Inport
  Area : Constant  Value=2.58
  Cd : Constant  Value=0.35
  Gain : Gain  Gain=0.5
  Square : Math  Operator=square
  Subtract : Sum  Inputs=+-
  product : Product  Inputs=4
  rho : Constant  Value=1.18
  v_wind : Constant  Value=0
  F_aero : Outport
  wires:
  Cd/1 -> product/2
  velocity/1 -> Subtract/1
  v_wind/1 -> Subtract/2
  product/1 -> F_aero/1
  rho/1 -> Gain/1
  Area/1 -> product/1
  Gain/1 -> product/3
  Subtract/1 -> Square/1
  Square/1 -> product/4

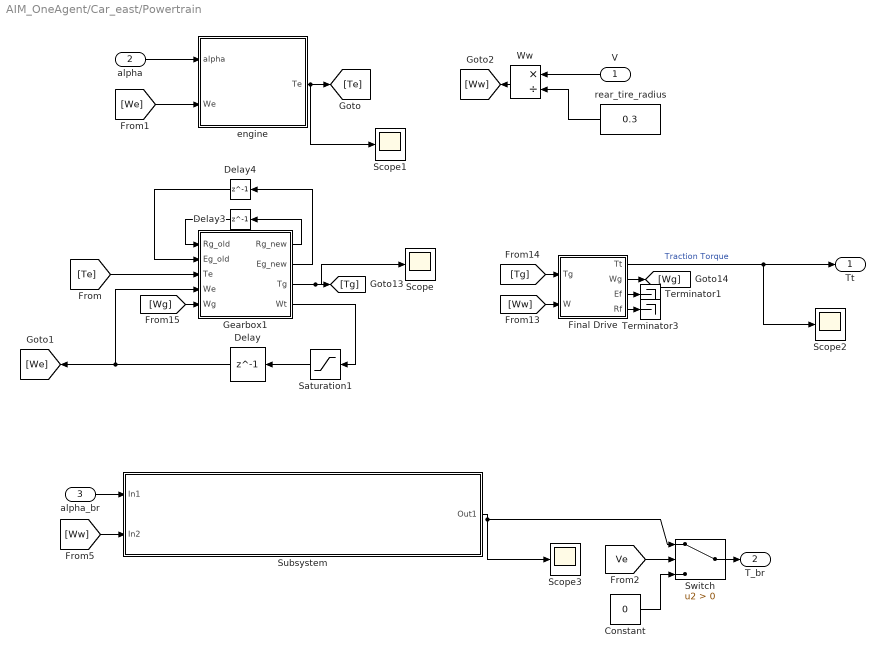
== system AIM_OneAgent/Car_east/Powertrain ==
  V : Inport
  alpha : Inport  Port=2
  alpha_br : Inport  Port=3
  Constant : Constant  Value=0
  Delay : Delay  DelayLength=1  InitialCondition=0
  Delay3 : Delay  DelayLength=1  InitialCondition=2.8
  Delay4 : Delay  DelayLength=1  InitialCondition=0.94
  Final Drive : Subsystem
  Gearbox1 : MATLAB Function  TreatAsAtomicUnit=on
  Saturation1 : Saturate  UpperLimit=6000*(pi/30)  LowerLimit=500*(pi/30)  LinearizeAsGain=off
  Scope{,1..3} (4 alike) : Scope
  Subsystem : Subsystem
  Switch : Switch  Criteria=u2 > Threshold  SaturateOnIntegerOverflow=off  InputSameDT=off
  Terminator1 : Terminator
  Terminator3 : Terminator
  Ww : Product  Inputs=*/  RndMeth=Zero  SaturateOnIntegerOverflow=on
  engine : Subsystem
  rear_tire_radius : Constant  Value=0.3
  Tt : Outport
  T_br : Outport  Port=2
  wires:
  rear_tire_radius/1 -> Ww/2
  alpha/1 -> engine/1(alpha)
  [We] -> engine/2(We)
  V/1 -> Ww/1
  Ww/1 -> [Ww]
  alpha_br/1 -> Subsystem/1(In1)
  [Ww] -> Subsystem/2(In2)
  Gearbox1/2(Eg_new) -> Delay4/1
  Gearbox1/1(Rg_new) -> Delay3/1
  Delay4/1 -> Gearbox1/2(Eg_old)
  Gearbox1/3(Tg) -> Scope/1, [Tg]
  Delay3/1 -> Gearbox1/1(Rg_old)
  Saturation1/1 -> Delay/1
  Delay/1 -> [We], Gearbox1/4(We)
  [Wg] -> Gearbox1/5(Wg)
  [Te] -> Gearbox1/3(Te)
  Gearbox1/4(Wt) -> Saturation1/1
  Final Drive/1(Tt) -> Scope2/1, Tt/1  "Traction Torque"
  Final Drive/3(Ef) -> Terminator1/1
  Final Drive/2(Wg) -> [Wg]
  Final Drive/4(Rf) -> Terminator3/1
  [Tg] -> Final Drive/1(Tg)
  [Ww] -> Final Drive/2(W)
  engine/1(Te) -> Scope1/1, [Te]
  [Ve] -> Switch/2
  Subsystem/1(Out1) -> Switch/1, Scope3/1
  Switch/1 -> T_br/1
  Constant/1 -> Switch/3

== system AIM_OneAgent/Car_east/Rx ==
  C : Constant  Value=0.01
  g : Constant  Value=9.8
  mass : Constant  Value=1800
  product : Product  Inputs=3
  Rx : Outport
  wires:
  mass/1 -> product/1
  g/1 -> product/2
  C/1 -> product/3
  product/1 -> Rx/1

== system AIM_OneAgent/Car_north/F_aero ==
  velocity : Inport
  Area : Constant  Value=2.58
  Cd : Constant  Value=0.35
  Gain : Gain  Gain=0.5
  Square : Math  Operator=square
  Subtract : Sum  Inputs=+-
  product : Product  Inputs=4
  rho : Constant  Value=1.18
  v_wind : Constant  Value=0
  F_aero : Outport
  wires:
  Cd/1 -> product/2
  velocity/1 -> Subtract/1
  v_wind/1 -> Subtract/2
  product/1 -> F_aero/1
  rho/1 -> Gain/1
  Area/1 -> product/1
  Gain/1 -> product/3
  Subtract/1 -> Square/1
  Square/1 -> product/4

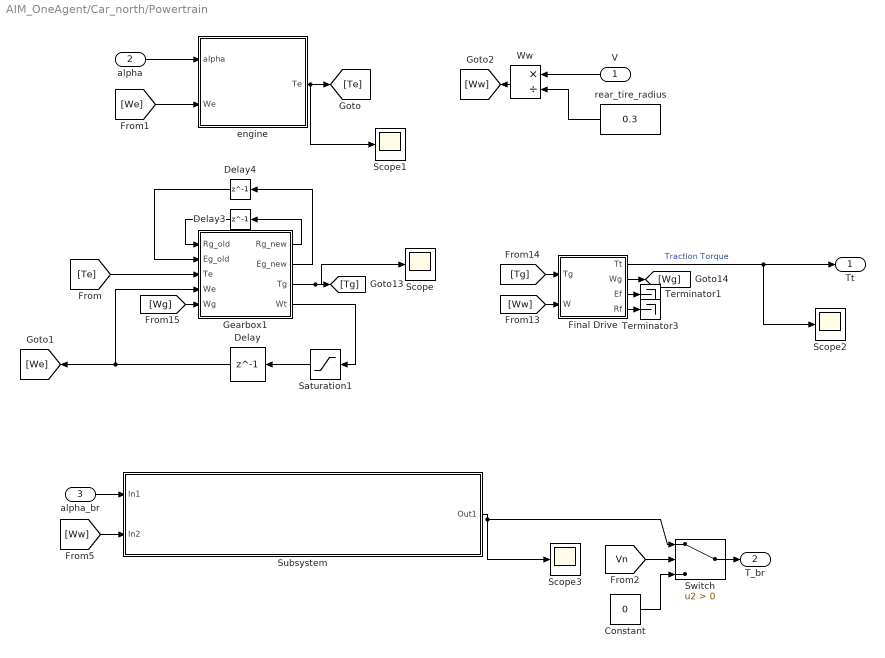
== system AIM_OneAgent/Car_north/Powertrain ==
  V : Inport
  alpha : Inport  Port=2
  alpha_br : Inport  Port=3
  Constant : Constant  Value=0
  Delay : Delay  DelayLength=1  InitialCondition=0
  Delay3 : Delay  DelayLength=1  InitialCondition=2.8
  Delay4 : Delay  DelayLength=1  InitialCondition=0.94
  Final Drive : Subsystem
  Gearbox1 : MATLAB Function  TreatAsAtomicUnit=on
  Saturation1 : Saturate  UpperLimit=6000*(pi/30)  LowerLimit=500*(pi/30)  LinearizeAsGain=off
  Scope{,1..3} (4 alike) : Scope
  Subsystem : Subsystem
  Switch : Switch  Criteria=u2 > Threshold  SaturateOnIntegerOverflow=off  InputSameDT=off
  Terminator1 : Terminator
  Terminator3 : Terminator
  Ww : Product  Inputs=*/  RndMeth=Zero  SaturateOnIntegerOverflow=on
  engine : Subsystem
  rear_tire_radius : Constant  Value=0.3
  Tt : Outport
  T_br : Outport  Port=2
  wires:
  rear_tire_radius/1 -> Ww/2
  alpha/1 -> engine/1(alpha)
  [We] -> engine/2(We)
  V/1 -> Ww/1
  Ww/1 -> [Ww]
  alpha_br/1 -> Subsystem/1(In1)
  [Ww] -> Subsystem/2(In2)
  Gearbox1/2(Eg_new) -> Delay4/1
  Gearbox1/1(Rg_new) -> Delay3/1
  Delay4/1 -> Gearbox1/2(Eg_old)
  Gearbox1/3(Tg) -> Scope/1, [Tg]
  Delay3/1 -> Gearbox1/1(Rg_old)
  Saturation1/1 -> Delay/1
  Delay/1 -> [We], Gearbox1/4(We)
  [Wg] -> Gearbox1/5(Wg)
  [Te] -> Gearbox1/3(Te)
  Gearbox1/4(Wt) -> Saturation1/1
  Final Drive/1(Tt) -> Scope2/1, Tt/1  "Traction Torque"
  Final Drive/3(Ef) -> Terminator1/1
  Final Drive/2(Wg) -> [Wg]
  Final Drive/4(Rf) -> Terminator3/1
  [Tg] -> Final Drive/1(Tg)
  [Ww] -> Final Drive/2(W)
  engine/1(Te) -> Scope1/1, [Te]
  [Vn] -> Switch/2
  Subsystem/1(Out1) -> Switch/1, Scope3/1
  Switch/1 -> T_br/1
  Constant/1 -> Switch/3

== system AIM_OneAgent/Car_north/Rx ==
  C : Constant  Value=0.01
  g : Constant  Value=9.8
  mass : Constant  Value=1800
  product : Product  Inputs=3
  Rx : Outport
  wires:
  mass/1 -> product/1
  g/1 -> product/2
  C/1 -> product/3
  product/1 -> Rx/1

== system AIM_OneAgent/Car_south/F_aero ==
  velocity : Inport
  Area : Constant  Value=2.58
  Cd : Constant  Value=0.35
  Gain : Gain  Gain=0.5
  Square : Math  Operator=square
  Subtract : Sum  Inputs=+-
  product : Product  Inputs=4
  rho : Constant  Value=1.18
  v_wind : Constant  Value=0
  F_aero : Outport
  wires:
  Cd/1 -> product/2
  velocity/1 -> Subtract/1
  v_wind/1 -> Subtract/2
  product/1 -> F_aero/1
  rho/1 -> Gain/1
  Area/1 -> product/1
  Gain/1 -> product/3
  Subtract/1 -> Square/1
  Square/1 -> product/4

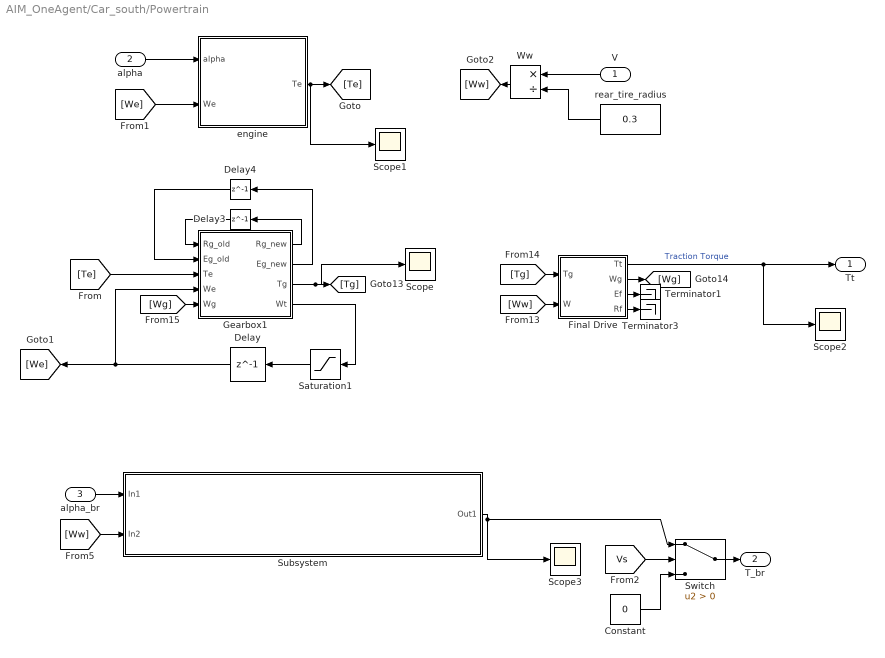
== system AIM_OneAgent/Car_south/Powertrain ==
  V : Inport
  alpha : Inport  Port=2
  alpha_br : Inport  Port=3
  Constant : Constant  Value=0
  Delay : Delay  DelayLength=1  InitialCondition=0
  Delay3 : Delay  DelayLength=1  InitialCondition=2.8
  Delay4 : Delay  DelayLength=1  InitialCondition=0.94
  Final Drive : Subsystem
  Gearbox1 : MATLAB Function  TreatAsAtomicUnit=on
  Saturation1 : Saturate  UpperLimit=6000*(pi/30)  LowerLimit=500*(pi/30)  LinearizeAsGain=off
  Scope{,1..3} (4 alike) : Scope
  Subsystem : Subsystem
  Switch : Switch  Criteria=u2 > Threshold  SaturateOnIntegerOverflow=off  InputSameDT=off
  Terminator1 : Terminator
  Terminator3 : Terminator
  Ww : Product  Inputs=*/  RndMeth=Zero  SaturateOnIntegerOverflow=on
  engine : Subsystem
  rear_tire_radius : Constant  Value=0.3
  Tt : Outport
  T_br : Outport  Port=2
  wires:
  rear_tire_radius/1 -> Ww/2
  alpha/1 -> engine/1(alpha)
  [We] -> engine/2(We)
  V/1 -> Ww/1
  Ww/1 -> [Ww]
  alpha_br/1 -> Subsystem/1(In1)
  [Ww] -> Subsystem/2(In2)
  Gearbox1/2(Eg_new) -> Delay4/1
  Gearbox1/1(Rg_new) -> Delay3/1
  Delay4/1 -> Gearbox1/2(Eg_old)
  Gearbox1/3(Tg) -> Scope/1, [Tg]
  Delay3/1 -> Gearbox1/1(Rg_old)
  Saturation1/1 -> Delay/1
  Delay/1 -> [We], Gearbox1/4(We)
  [Wg] -> Gearbox1/5(Wg)
  [Te] -> Gearbox1/3(Te)
  Gearbox1/4(Wt) -> Saturation1/1
  Final Drive/1(Tt) -> Scope2/1, Tt/1  "Traction Torque"
  Final Drive/3(Ef) -> Terminator1/1
  Final Drive/2(Wg) -> [Wg]
  Final Drive/4(Rf) -> Terminator3/1
  [Tg] -> Final Drive/1(Tg)
  [Ww] -> Final Drive/2(W)
  engine/1(Te) -> Scope1/1, [Te]
  [Vs] -> Switch/2
  Subsystem/1(Out1) -> Switch/1, Scope3/1
  Switch/1 -> T_br/1
  Constant/1 -> Switch/3

== system AIM_OneAgent/Car_south/Rx ==
  C : Constant  Value=0.01
  g : Constant  Value=9.8
  mass : Constant  Value=1800
  product : Product  Inputs=3
  Rx : Outport
  wires:
  mass/1 -> product/1
  g/1 -> product/2
  C/1 -> product/3
  product/1 -> Rx/1

== system AIM_OneAgent/Car_west/F_aero ==
  velocity : Inport
  Area : Constant  Value=2.58
  Cd : Constant  Value=0.35
  Gain : Gain  Gain=0.5
  Square : Math  Operator=square
  Subtract : Sum  Inputs=+-
  product : Product  Inputs=4
  rho : Constant  Value=1.18
  v_wind : Constant  Value=0
  F_aero : Outport
  wires:
  Cd/1 -> product/2
  velocity/1 -> Subtract/1
  v_wind/1 -> Subtract/2
  product/1 -> F_aero/1
  rho/1 -> Gain/1
  Area/1 -> product/1
  Gain/1 -> product/3
  Subtract/1 -> Square/1
  Square/1 -> product/4

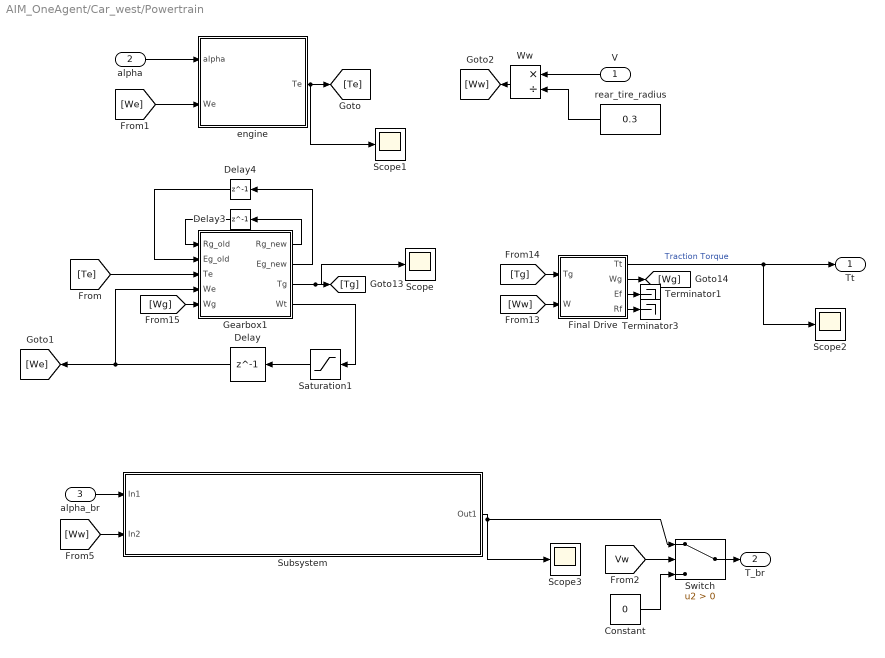
== system AIM_OneAgent/Car_west/Powertrain ==
  V : Inport
  alpha : Inport  Port=2
  alpha_br : Inport  Port=3
  Constant : Constant  Value=0
  Delay : Delay  DelayLength=1  InitialCondition=0
  Delay3 : Delay  DelayLength=1  InitialCondition=2.8
  Delay4 : Delay  DelayLength=1  InitialCondition=0.94
  Final Drive : Subsystem
  Gearbox1 : MATLAB Function  TreatAsAtomicUnit=on
  Saturation1 : Saturate  UpperLimit=6000*(pi/30)  LowerLimit=500*(pi/30)  LinearizeAsGain=off
  Scope{,1..3} (4 alike) : Scope
  Subsystem : Subsystem
  Switch : Switch  Criteria=u2 > Threshold  SaturateOnIntegerOverflow=off  InputSameDT=off
  Terminator1 : Terminator
  Terminator3 : Terminator
  Ww : Product  Inputs=*/  RndMeth=Zero  SaturateOnIntegerOverflow=on
  engine : Subsystem
  rear_tire_radius : Constant  Value=0.3
  Tt : Outport
  T_br : Outport  Port=2
  wires:
  rear_tire_radius/1 -> Ww/2
  alpha/1 -> engine/1(alpha)
  [We] -> engine/2(We)
  V/1 -> Ww/1
  Ww/1 -> [Ww]
  alpha_br/1 -> Subsystem/1(In1)
  [Ww] -> Subsystem/2(In2)
  Gearbox1/2(Eg_new) -> Delay4/1
  Gearbox1/1(Rg_new) -> Delay3/1
  Delay4/1 -> Gearbox1/2(Eg_old)
  Gearbox1/3(Tg) -> Scope/1, [Tg]
  Delay3/1 -> Gearbox1/1(Rg_old)
  Saturation1/1 -> Delay/1
  Delay/1 -> [We], Gearbox1/4(We)
  [Wg] -> Gearbox1/5(Wg)
  [Te] -> Gearbox1/3(Te)
  Gearbox1/4(Wt) -> Saturation1/1
  Final Drive/1(Tt) -> Scope2/1, Tt/1  "Traction Torque"
  Final Drive/3(Ef) -> Terminator1/1
  Final Drive/2(Wg) -> [Wg]
  Final Drive/4(Rf) -> Terminator3/1
  [Tg] -> Final Drive/1(Tg)
  [Ww] -> Final Drive/2(W)
  engine/1(Te) -> Scope1/1, [Te]
  [Vw] -> Switch/2
  Subsystem/1(Out1) -> Switch/1, Scope3/1
  Switch/1 -> T_br/1
  Constant/1 -> Switch/3

== system AIM_OneAgent/Car_west/Rx ==
  C : Constant  Value=0.01
  g : Constant  Value=9.8
  mass : Constant  Value=1800
  product : Product  Inputs=3
  Rx : Outport
  wires:
  mass/1 -> product/1
  g/1 -> product/2
  C/1 -> product/3
  product/1 -> Rx/1

== system AIM_OneAgent/Car_east/Powertrain/Final Drive ==
  Tg : Inport
  W : Inport  Port=2
  Final drive efficiency : Constant
  Final drive ratio : Constant  Value=3.64
  Product : Product  Inputs=3
  Product1 : Product
  Tt : Outport  VectorParamsAs1DForOutWhenUnconnected=off
  Wg : Outport  Port=2  VectorParamsAs1DForOutWhenUnconnected=off
  Ef : Outport  Port=3  VectorParamsAs1DForOutWhenUnconnected=off
  Rf : Outport  Port=4  VectorParamsAs1DForOutWhenUnconnected=off
  wires:
  Product/1 -> Tt/1
  Final drive ratio/1 -> Rf/1, Product/3, Product1/1
  Tg/1 -> Product/2
  Product1/1 -> Wg/1
  W/1 -> Product1/2
  Final drive efficiency/1 -> Ef/1, Product/1

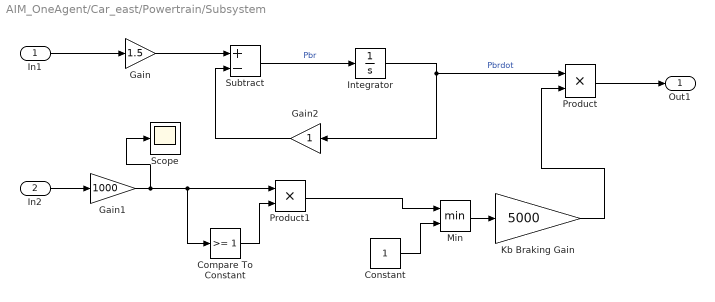
== system AIM_OneAgent/Car_east/Powertrain/Subsystem ==
  In1 : Inport
  In2 : Inport  Port=2
  Compare To Constant : simulink/Logic and Bit Operations/Compare To Constant  relop=>=  const=1  OutDataTypeStr=boolean
  Constant : Constant
  Gain : Gain  Gain=1.5
  Gain1 : Gain  Gain=1000
  Gain2 : Gain
  Integrator : Integrator
  Kb Braking Gain : Gain  Gain=5000
  Min : MinMax  Inputs=2
  Product : Product
  Product1 : Product
  Scope : Scope
  Subtract : Sum  Inputs=+-
  Out1 : Outport
  wires:
  Gain1/1 -> Scope/1, Compare To Constant/1, Product1/1
  Min/1 -> Kb Braking Gain/1
  Subtract/1 -> Integrator/1  "Pbr"
  Gain/1 -> Subtract/1
  In2/1 -> Gain1/1
  In1/1 -> Gain/1
  Integrator/1 -> Product/1, Gain2/1  "Pbrdot"
  Product1/1 -> Min/1
  Gain2/1 -> Subtract/2
  Compare To Constant/1 -> Product1/2
  Kb Braking Gain/1 -> Product/2
  Constant/1 -> Min/2
  Product/1 -> Out1/1

== system AIM_OneAgent/Car_east/Powertrain/engine ==
  alpha : Inport
  We : Inport  Port=2
  engine : Subsystem
  Te : Outport
  wires:
  alpha/1 -> engine/1(alpha)
  We/1 -> engine/2(We)
  engine/1(Te) -> Te/1

== system AIM_OneAgent/Car_north/Powertrain/Final Drive ==
  Tg : Inport
  W : Inport  Port=2
  Final drive efficiency : Constant
  Final drive ratio : Constant  Value=3.64
  Product : Product  Inputs=3
  Product1 : Product
  Tt : Outport  VectorParamsAs1DForOutWhenUnconnected=off
  Wg : Outport  Port=2  VectorParamsAs1DForOutWhenUnconnected=off
  Ef : Outport  Port=3  VectorParamsAs1DForOutWhenUnconnected=off
  Rf : Outport  Port=4  VectorParamsAs1DForOutWhenUnconnected=off
  wires:
  Product/1 -> Tt/1
  Final drive ratio/1 -> Rf/1, Product/3, Product1/1
  Tg/1 -> Product/2
  Product1/1 -> Wg/1
  W/1 -> Product1/2
  Final drive efficiency/1 -> Ef/1, Product/1

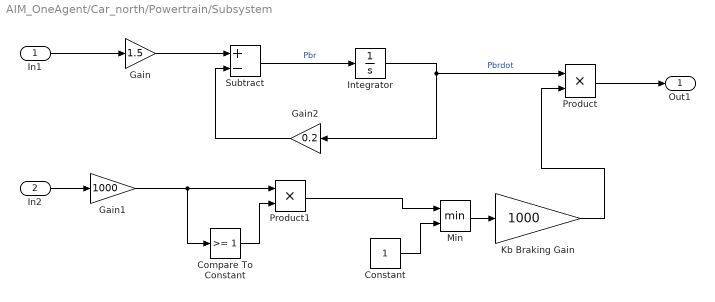
== system AIM_OneAgent/Car_north/Powertrain/Subsystem ==
  In1 : Inport
  In2 : Inport  Port=2
  Compare To Constant : simulink/Logic and Bit Operations/Compare To Constant  relop=>=  const=1  OutDataTypeStr=boolean
  Constant : Constant
  Gain : Gain  Gain=1.5
  Gain1 : Gain  Gain=1000
  Gain2 : Gain  Gain=0.2
  Integrator : Integrator
  Kb Braking Gain : Gain  Gain=1000
  Min : MinMax  Inputs=2
  Product : Product
  Product1 : Product
  Subtract : Sum  Inputs=+-
  Out1 : Outport
  wires:
  Gain1/1 -> Compare To Constant/1, Product1/1
  Min/1 -> Kb Braking Gain/1
  Subtract/1 -> Integrator/1  "Pbr"
  Gain/1 -> Subtract/1
  In2/1 -> Gain1/1
  In1/1 -> Gain/1
  Integrator/1 -> Product/1, Gain2/1  "Pbrdot"
  Product1/1 -> Min/1
  Gain2/1 -> Subtract/2
  Compare To Constant/1 -> Product1/2
  Kb Braking Gain/1 -> Product/2
  Constant/1 -> Min/2
  Product/1 -> Out1/1

== system AIM_OneAgent/Car_north/Powertrain/engine ==
  alpha : Inport
  We : Inport  Port=2
  engine : Subsystem
  Te : Outport
  wires:
  alpha/1 -> engine/1(alpha)
  We/1 -> engine/2(We)
  engine/1(Te) -> Te/1

== system AIM_OneAgent/Car_south/Powertrain/Final Drive ==
  Tg : Inport
  W : Inport  Port=2
  Final drive efficiency : Constant
  Final drive ratio : Constant  Value=3.64
  Product : Product  Inputs=3
  Product1 : Product
  Tt : Outport  VectorParamsAs1DForOutWhenUnconnected=off
  Wg : Outport  Port=2  VectorParamsAs1DForOutWhenUnconnected=off
  Ef : Outport  Port=3  VectorParamsAs1DForOutWhenUnconnected=off
  Rf : Outport  Port=4  VectorParamsAs1DForOutWhenUnconnected=off
  wires:
  Product/1 -> Tt/1
  Final drive ratio/1 -> Rf/1, Product/3, Product1/1
  Tg/1 -> Product/2
  Product1/1 -> Wg/1
  W/1 -> Product1/2
  Final drive efficiency/1 -> Ef/1, Product/1

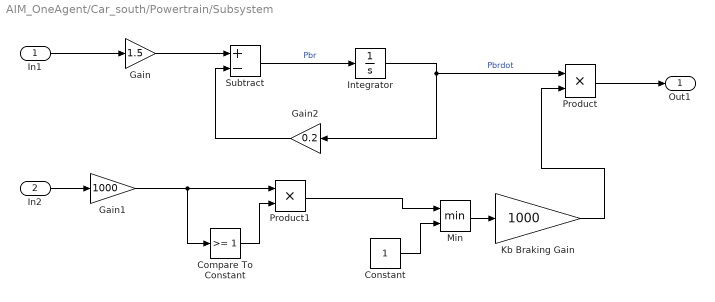
== system AIM_OneAgent/Car_south/Powertrain/Subsystem ==
  In1 : Inport
  In2 : Inport  Port=2
  Compare To Constant : simulink/Logic and Bit Operations/Compare To Constant  relop=>=  const=1  OutDataTypeStr=boolean
  Constant : Constant
  Gain : Gain  Gain=1.5
  Gain1 : Gain  Gain=1000
  Gain2 : Gain  Gain=0.2
  Integrator : Integrator
  Kb Braking Gain : Gain  Gain=1000
  Min : MinMax  Inputs=2
  Product : Product
  Product1 : Product
  Subtract : Sum  Inputs=+-
  Out1 : Outport
  wires:
  Gain1/1 -> Compare To Constant/1, Product1/1
  Min/1 -> Kb Braking Gain/1
  Subtract/1 -> Integrator/1  "Pbr"
  Gain/1 -> Subtract/1
  In2/1 -> Gain1/1
  In1/1 -> Gain/1
  Integrator/1 -> Product/1, Gain2/1  "Pbrdot"
  Product1/1 -> Min/1
  Gain2/1 -> Subtract/2
  Compare To Constant/1 -> Product1/2
  Kb Braking Gain/1 -> Product/2
  Constant/1 -> Min/2
  Product/1 -> Out1/1

== system AIM_OneAgent/Car_south/Powertrain/engine ==
  alpha : Inport
  We : Inport  Port=2
  engine : Subsystem
  Te : Outport
  wires:
  alpha/1 -> engine/1(alpha)
  We/1 -> engine/2(We)
  engine/1(Te) -> Te/1

== system AIM_OneAgent/Car_west/Powertrain/Final Drive ==
  Tg : Inport
  W : Inport  Port=2
  Final drive efficiency : Constant
  Final drive ratio : Constant  Value=3.64
  Product : Product  Inputs=3
  Product1 : Product
  Tt : Outport  VectorParamsAs1DForOutWhenUnconnected=off
  Wg : Outport  Port=2  VectorParamsAs1DForOutWhenUnconnected=off
  Ef : Outport  Port=3  VectorParamsAs1DForOutWhenUnconnected=off
  Rf : Outport  Port=4  VectorParamsAs1DForOutWhenUnconnected=off
  wires:
  Product/1 -> Tt/1
  Final drive ratio/1 -> Rf/1, Product/3, Product1/1
  Tg/1 -> Product/2
  Product1/1 -> Wg/1
  W/1 -> Product1/2
  Final drive efficiency/1 -> Ef/1, Product/1

== system AIM_OneAgent/Car_west/Powertrain/Subsystem ==
  In1 : Inport
  In2 : Inport  Port=2
  Compare To Constant : simulink/Logic and Bit Operations/Compare To Constant  relop=>=  const=1  OutDataTypeStr=boolean
  Constant : Constant
  Gain : Gain  Gain=1.5
  Gain1 : Gain  Gain=1000
  Gain2 : Gain  Gain=0.2
  Integrator : Integrator
  Kb Braking Gain : Gain  Gain=1000
  Min : MinMax  Inputs=2
  Product : Product
  Product1 : Product
  Subtract : Sum  Inputs=+-
  Out1 : Outport
  wires:
  Gain1/1 -> Compare To Constant/1, Product1/1
  Min/1 -> Kb Braking Gain/1
  Subtract/1 -> Integrator/1  "Pbr"
  Gain/1 -> Subtract/1
  In2/1 -> Gain1/1
  In1/1 -> Gain/1
  Integrator/1 -> Product/1, Gain2/1  "Pbrdot"
  Product1/1 -> Min/1
  Gain2/1 -> Subtract/2
  Compare To Constant/1 -> Product1/2
  Kb Braking Gain/1 -> Product/2
  Constant/1 -> Min/2
  Product/1 -> Out1/1

== system AIM_OneAgent/Car_west/Powertrain/engine ==
  alpha : Inport
  We : Inport  Port=2
  engine : Subsystem
  Te : Outport
  wires:
  alpha/1 -> engine/1(alpha)
  We/1 -> engine/2(We)
  engine/1(Te) -> Te/1

== system AIM_OneAgent/Car_east/Powertrain/engine/engine ==
  alpha : Inport
  We : Inport  Port=2
  MATLAB Function : MATLAB Function  TreatAsAtomicUnit=on
  Pmax : Constant  Value=100e3
  Wo : Constant  Value=5100 * (pi/30)
  Te : Outport
  wires:
  We/1 -> MATLAB Function/4(We)
  Wo/1 -> MATLAB Function/3(Wo)
  Pmax/1 -> MATLAB Function/2(Pmax)
  alpha/1 -> MATLAB Function/1(alpha)
  MATLAB Function/1(Te) -> Te/1

== system AIM_OneAgent/Car_north/Powertrain/engine/engine ==
  alpha : Inport
  We : Inport  Port=2
  MATLAB Function : MATLAB Function  TreatAsAtomicUnit=on
  Pmax : Constant  Value=100e3
  Wo : Constant  Value=5100 * (pi/30)
  Te : Outport
  wires:
  We/1 -> MATLAB Function/4(We)
  Wo/1 -> MATLAB Function/3(Wo)
  Pmax/1 -> MATLAB Function/2(Pmax)
  alpha/1 -> MATLAB Function/1(alpha)
  MATLAB Function/1(Te) -> Te/1

== system AIM_OneAgent/Car_south/Powertrain/engine/engine ==
  alpha : Inport
  We : Inport  Port=2
  MATLAB Function : MATLAB Function  TreatAsAtomicUnit=on
  Pmax : Constant  Value=100e3
  Wo : Constant  Value=5100 * (pi/30)
  Te : Outport
  wires:
  We/1 -> MATLAB Function/4(We)
  Wo/1 -> MATLAB Function/3(Wo)
  Pmax/1 -> MATLAB Function/2(Pmax)
  alpha/1 -> MATLAB Function/1(alpha)
  MATLAB Function/1(Te) -> Te/1

== system AIM_OneAgent/Car_west/Powertrain/engine/engine ==
  alpha : Inport
  We : Inport  Port=2
  MATLAB Function : MATLAB Function  TreatAsAtomicUnit=on
  Pmax : Constant  Value=100e3
  Wo : Constant  Value=5100 * (pi/30)
  Te : Outport
  wires:
  We/1 -> MATLAB Function/4(We)
  Wo/1 -> MATLAB Function/3(Wo)
  Pmax/1 -> MATLAB Function/2(Pmax)
  alpha/1 -> MATLAB Function/1(alpha)
  MATLAB Function/1(Te) -> Te/1

== matlab function AIM_OneAgent/Car_north/MATLAB Function ==
  data: u input; Ut output; Ub output
function [Ut,Ub] = fcn(u)

 if(u>-0.05 && u<0)
      Ub=0;
      Ut=0;
 elseif(u<-0.05 && u<0)
 Ut=0;
 Ub=-u;
  else
 Ut=u;
 Ub=0;
%  end
 end

== matlab function AIM_OneAgent/Car_north/MATLAB Function1 ==
  data: F_aero input; a output; Rx input; Tt input; T_br input
function a = fcn(F_aero , Rx , Tt , T_br)

m = 1400;
Iw = 1.5;
reff = 0.32;

% a = (Tt - T_br - ( (F_aero + Rx)*reff) ) / (m*reff + Iw/reff);

M = (m*reff)+(Iw/reff);
a = (Tt-T_br-reff*(F_aero+Rx))/M;

end

== matlab function AIM_OneAgent/visualization ==
  data: pe input; ps input; pn input; pw input; collided output
function collided = drawEnvironment(pe, ps, pn,pw)
collided = false;
coder.extrinsic("plotEnvironment");
collided = plotEnvironment(pe,ps,pn,pw);
